simulink library "dlbsBlockSlice"  (R2025b)
settings: Solver=VariableStepAuto  StartTime=0.0  StopTime=10.0  RelTol=1e-3
libraries: dlbsBlockExtractGradientGF x9, dlbsBlockParametrizedSelector x9, dlbsBlockInsertGradientGF x3
settings Model: Creator=lt6037  LastModifiedBy=lt6037

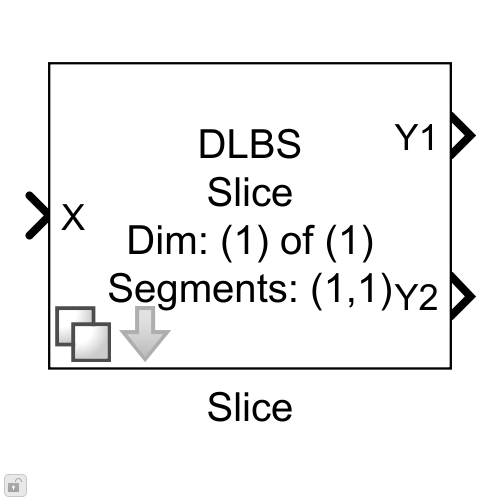
[thumbnail: Simulink's stored preview of the top-level diagram]
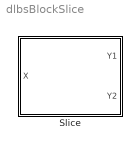
== system dlbsBlockSlice ==
  Slice : Subsystem  Variant=on  mask{n_out=2, all_dims=1, dim=1, s1=1, s2=1, s3=1, s4=1}
      mask prompts: n_out "Number of Inputs"; all_dims "Number of Dimensions"; dim "Working Dimension"; s1 "Length of Slice 1"; s2 "Length of Slice 2"; s3 "Length of Slice 3"; s4 "Length of Slice 4"
      mask help:
      | Slices an input tensor into multiple outputs along a selected working dimension. The user must specify slice lengths for each active output, because these lengths are required to concatenate output gradients back into the input gradient.
      | The last tensor dimension must not be of size 1. If the last dimension would be 1, reduce ALL_DIMS by 1 and omit that trailing singleton dimension. This avoids Simulink implicitly dropping a singleton final dimension.
      mask Help: web("dlbsHelpBlockSlice.html")
      mask DialogControl Container3 Prompt: Last Indecies of Slices
      mask Display:
      | m = Simulink.Mask.get(gcb);
      | dim = m.getParameter("dim").Value;
      | all_dims = m.getParameter("all_dims").Value;
      | n_out = str2double(m.getParameter("n_out").Value);
      | 
      | lines = string.empty;
      | 
      | lines(end+1) = "DLBS";
      | lines(end+1) = "Slice";
      | lines(end+1) = sprintf("Dim: (%s) of (%s)",dim, all_dims);
      | 
      | for n = 1:n_out
      |     s(n) = string(m.getParameter(sprintf("s%d",n)).Value);
      | end
      | 
      | lines(end+1) = sprintf("Segments: (%s)", strjoin(s,","));
      | 
      | disp(strjoin(lines,"\n"));

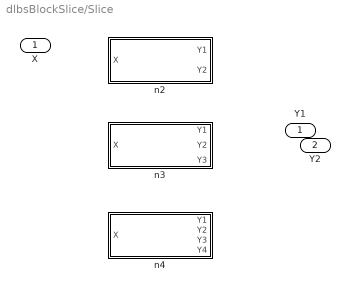
== system dlbsBlockSlice/Slice ==
  X : Inport
  n2 : Subsystem  VariantControl=n_out==2
  n3 : Subsystem  VariantControl=n_out==3
  n4 : Subsystem  VariantControl=n_out==4
  Y1 : Outport
  Y2 : Outport  Port=2

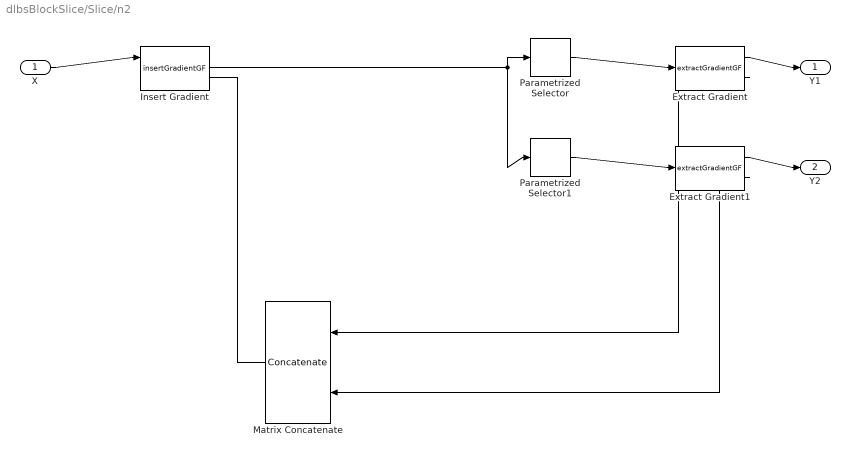
== system dlbsBlockSlice/Slice/n2 ==
  X : Inport
  Extract Gradient : dlbsBlockExtractGradientGF/extractGradientGF
  Extract Gradient1 : dlbsBlockExtractGradientGF/extractGradientGF
  Insert Gradient : dlbsBlockInsertGradientGF/insertGradientGF
  Matrix Concatenate : Concatenate  Mode=Multidimensional array  ConcatenateDimension=dim
  Parametrized Selector : dlbsBlockParametrizedSelector/Parametrized Selector  all_dims=all_dims  dim=dim  idx1=1  idx2=1+s1-1
  Parametrized Selector1 : dlbsBlockParametrizedSelector/Parametrized Selector  all_dims=all_dims  dim=dim  idx1=s1+1  idx2=s1+s2
  Y1 : Outport
  Y2 : Outport  Port=2
  wires:
  X/1 -> Insert Gradient/1
  Extract Gradient/1 -> Y1/1
  Extract Gradient1/1 -> Y2/1
  Parametrized Selector/1 -> Extract Gradient/1
  Parametrized Selector1/1 -> Extract Gradient1/1
  Insert Gradient/1 -> Parametrized Selector1/1, Parametrized Selector/1
  Matrix Concatenate/1 -> Insert Gradient/2
  Extract Gradient/2 -> Matrix Concatenate/1
  Extract Gradient1/2 -> Matrix Concatenate/2

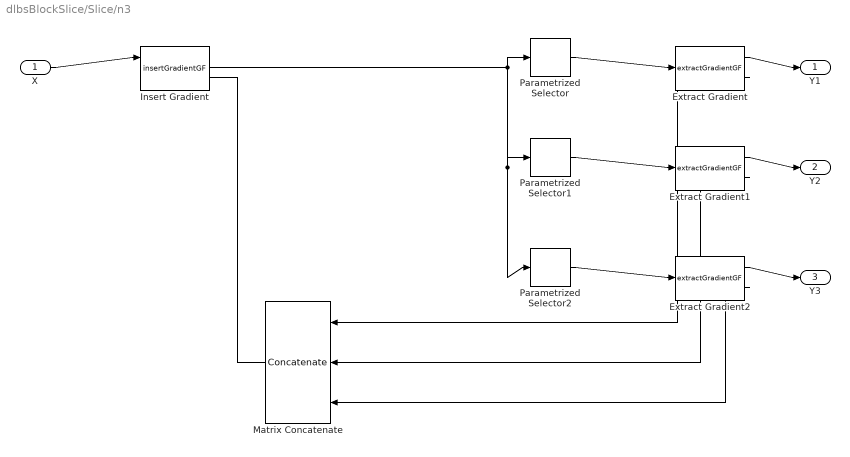
== system dlbsBlockSlice/Slice/n3 ==
  X : Inport
  Extract Gradient : dlbsBlockExtractGradientGF/extractGradientGF
  Extract Gradient1 : dlbsBlockExtractGradientGF/extractGradientGF
  Extract Gradient2 : dlbsBlockExtractGradientGF/extractGradientGF
  Insert Gradient : dlbsBlockInsertGradientGF/insertGradientGF
  Matrix Concatenate : Concatenate  NumInputs=3  Mode=Multidimensional array  ConcatenateDimension=dim
  Parametrized Selector : dlbsBlockParametrizedSelector/Parametrized Selector  all_dims=all_dims  dim=dim  idx1=1  idx2=1+s1-1
  Parametrized Selector1 : dlbsBlockParametrizedSelector/Parametrized Selector  all_dims=all_dims  dim=dim  idx1=s1+1  idx2=s1+s2
  Parametrized Selector2 : dlbsBlockParametrizedSelector/Parametrized Selector  all_dims=all_dims  dim=dim  idx1=s1+s2+1  idx2=s1+s2+s3
  Y1 : Outport
  Y2 : Outport  Port=2
  Y3 : Outport  Port=3
  wires:
  X/1 -> Insert Gradient/1
  Extract Gradient/1 -> Y1/1
  Extract Gradient1/1 -> Y2/1
  Extract Gradient2/1 -> Y3/1
  Parametrized Selector/1 -> Extract Gradient/1
  Parametrized Selector1/1 -> Extract Gradient1/1
  Parametrized Selector2/1 -> Extract Gradient2/1
  Insert Gradient/1 -> Parametrized Selector2/1, Parametrized Selector1/1, Parametrized Selector/1
  Matrix Concatenate/1 -> Insert Gradient/2
  Extract Gradient/2 -> Matrix Concatenate/1
  Extract Gradient1/2 -> Matrix Concatenate/2
  Extract Gradient2/2 -> Matrix Concatenate/3

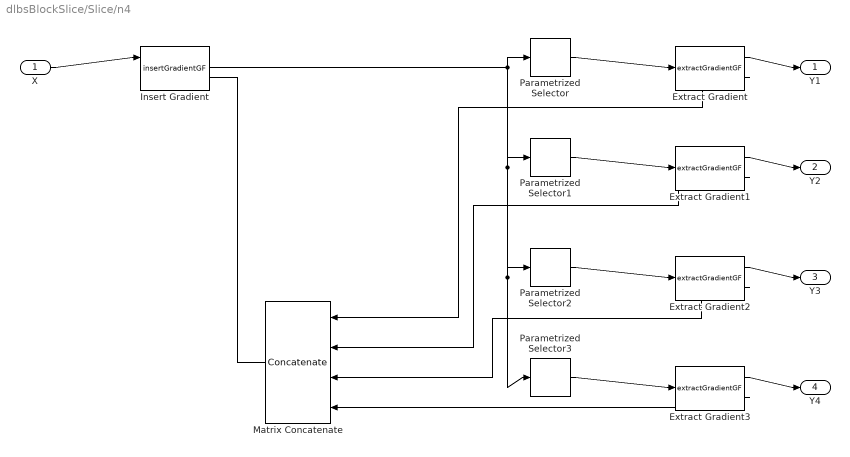
== system dlbsBlockSlice/Slice/n4 ==
  X : Inport
  Extract Gradient{,1..3} (4 alike) : dlbsBlockExtractGradientGF/extractGradientGF
  Insert Gradient : dlbsBlockInsertGradientGF/insertGradientGF
  Matrix Concatenate : Concatenate  NumInputs=4  Mode=Multidimensional array  ConcatenateDimension=dim
  Parametrized Selector : dlbsBlockParametrizedSelector/Parametrized Selector  all_dims=all_dims  dim=dim  idx1=1  idx2=1+s1-1
  Parametrized Selector1 : dlbsBlockParametrizedSelector/Parametrized Selector  all_dims=all_dims  dim=dim  idx1=s1+1  idx2=s1+s2
  Parametrized Selector2 : dlbsBlockParametrizedSelector/Parametrized Selector  all_dims=all_dims  dim=dim  idx1=s1+s2+1  idx2=s1+s2+s3
  Parametrized Selector3 : dlbsBlockParametrizedSelector/Parametrized Selector  all_dims=all_dims  dim=dim  idx1=s1+s2+s3+1  idx2=s1+s2+s3+s4
  Y1 : Outport
  Y2 : Outport  Port=2
  Y3 : Outport  Port=3
  Y4 : Outport  Port=4
  wires:
  X/1 -> Insert Gradient/1
  Extract Gradient/1 -> Y1/1
  Extract Gradient1/1 -> Y2/1
  Extract Gradient2/1 -> Y3/1
  Extract Gradient3/1 -> Y4/1
  Parametrized Selector/1 -> Extract Gradient/1
  Parametrized Selector1/1 -> Extract Gradient1/1
  Parametrized Selector2/1 -> Extract Gradient2/1
  Parametrized Selector3/1 -> Extract Gradient3/1
  Insert Gradient/1 -> Parametrized Selector3/1, Parametrized Selector2/1, Parametrized Selector1/1, Parametrized Selector/1
  Matrix Concatenate/1 -> Insert Gradient/2
  Extract Gradient/2 -> Matrix Concatenate/1
  Extract Gradient1/2 -> Matrix Concatenate/2
  Extract Gradient2/2 -> Matrix Concatenate/3
  Extract Gradient3/2 -> Matrix Concatenate/4
